simulink model "Landing_Sim_1"  (R2025b)
settings: Solver=VariableStepAuto  StartTime=0.0  StopTime=25  RelTol=1e-3
libraries: aerolibanim x1
settings Model: Creator=James  LastModifiedBy=James

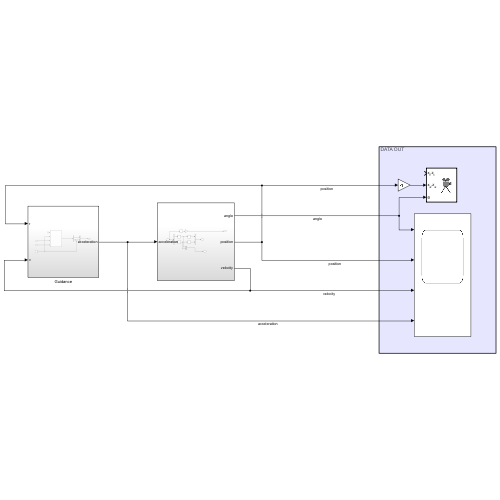
[thumbnail: Simulink's stored preview of the top-level diagram]
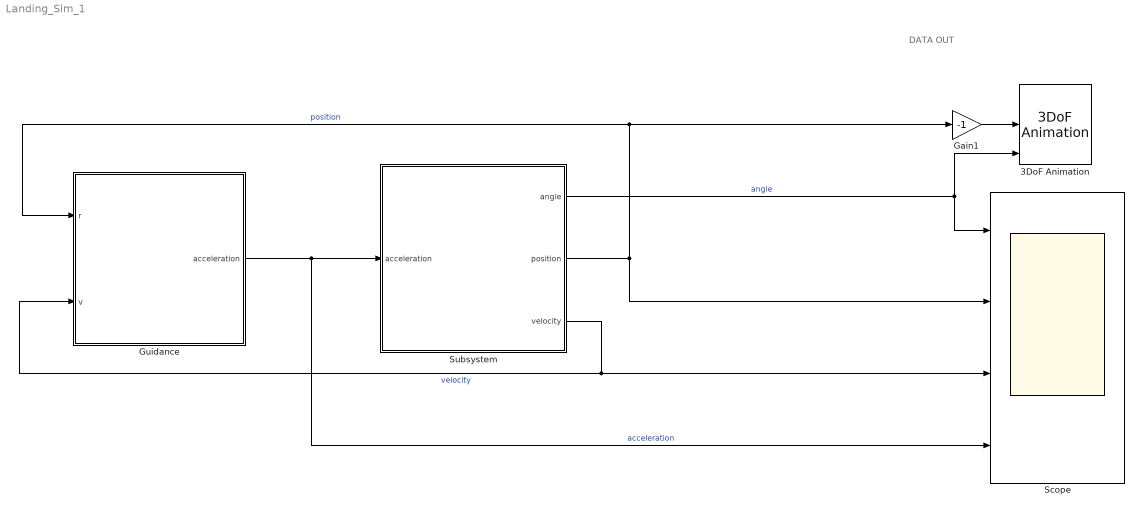
== system Landing_Sim_1 ==
  note: DATA OUT
  3DoF Animation : aerolibanim/3DoF Animation  u1=[0 5000 -2000 2000 -5050 -3050]  u2=0.05  u3=0.2  u5=Fixed position  u6=[50 150 0]  u7=30  u8=on
  Gain1 : Gain  Gain=-1
  Guidance : Subsystem
  Scope : Scope  NumInputPorts=4
      settings: ActiveDisplayYMinimum=-5.6195436966631531  ActiveDisplayYMaximum=10.364513599662731
  Subsystem : Subsystem
  wires:
  Gain1/1 -> 3DoF Animation/2
  Subsystem/3(velocity) -> Guidance/2(v), Scope/3  "velocity"
  Subsystem/2(position) -> Scope/2, Guidance/1(r), Gain1/1  "position"
  Subsystem/1(angle) -> Scope/1, 3DoF Animation/3  "angle"
  Guidance/1(acceleration) -> Scope/4, Subsystem/1(acceleration)  "acceleration"

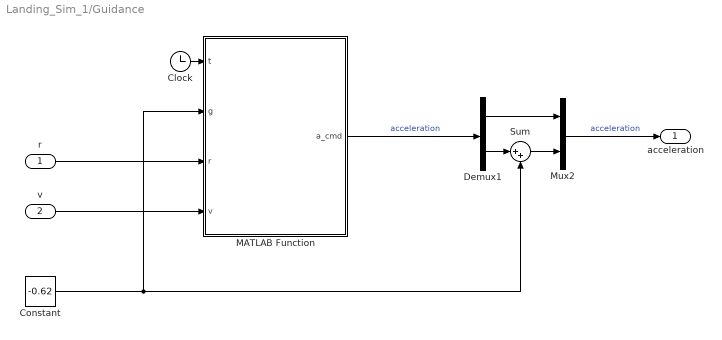
== system Landing_Sim_1/Guidance ==
  r : Inport
  v : Inport  Port=2
  Clock : Clock
  Constant : Constant  Value=-0.62
  Demux1 : Demux  Outputs=2
  MATLAB Function : MATLAB Function  TreatAsAtomicUnit=on
  Mux2 : Mux  Inputs=2
  Sum : Sum  Inputs=|++
  acceleration : Outport
  wires:
  Constant/1 -> Sum/2, MATLAB Function/2(g)
  Demux1/2 -> Sum/1
  MATLAB Function/1(a_cmd) -> Demux1/1  "acceleration"
  Demux1/1 -> Mux2/1
  Clock/1 -> MATLAB Function/1(t)
  Sum/1 -> Mux2/2
  Mux2/1 -> acceleration/1  "acceleration"
  r/1 -> MATLAB Function/3(r)
  v/1 -> MATLAB Function/4(v)

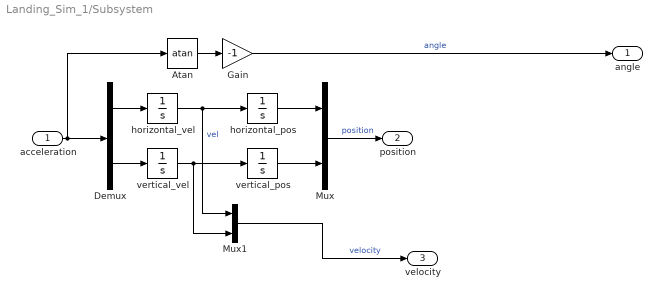
== system Landing_Sim_1/Subsystem ==
  acceleration : Inport
  Atan : Trigonometry  Operator=atan
  Demux : Demux  Outputs=2
  Gain : Gain  Gain=-1
  Mux : Mux  Inputs=2
  Mux1 : Mux  Inputs=2
  horizontal_pos : Integrator  InitialCondition=-200
  horizontal_vel : Integrator  InitialCondition=30
  vertical_pos : Integrator  InitialCondition=50
  vertical_vel : Integrator
  angle : Outport
  position : Outport  Port=2
  velocity : Outport  Port=3
  wires:
  horizontal_vel/1 -> Mux1/1, horizontal_pos/1  "vel"
  Mux/1 -> position/1  "position"
  vertical_pos/1 -> Mux/2
  vertical_vel/1 -> Mux1/2, vertical_pos/1
  Atan/1 -> Gain/1
  Demux/2 -> vertical_vel/1
  Demux/1 -> horizontal_vel/1
  horizontal_pos/1 -> Mux/1
  Mux1/1 -> velocity/1  "velocity"
  Gain/1 -> angle/1  "angle"
  acceleration/1 -> Atan/1, Demux/1

== matlab function Landing_Sim_1/Guidance/MATLAB Function ==
  data: t input; g input; a_cmd output; r input; v input
function a_cmd = guidance(t, g, r, v)
    a_max   = 50;
    r_f     = [0; 0];      % land at origin
    v_f     = [0; -0.1];   % gentle touchdown velocity
    t_land  = 13;          % total descent time (was t_a + t_f)
    tau_min = 0.25;

    tau = max(t_land - t, tau_min);

    ZEM = r_f - (r + v*tau + 0.5*g*tau^2);
    ZEV = v_f - (v + g*tau);
    a_cmd = (6/tau^2)*ZEM - (2/tau)*ZEV;

    n = norm(a_cmd);
    if n > a_max
        a_cmd = a_cmd * (a_max/n);
    end

    a_cycle = a_cmd/a_max;
end
